simulink model "BRO_piston_MOD_test"  (R2020b)
settings: Solver=FixedStepAuto  StartTime=0.0  StopTime=time_max  FixedStep=.1  RelTol=1e-3
values from neighbouring files (symbols this model uses):
  A_mem = 30    [BRO_parameters_MOD.m]    (also in Copy_of_BRO_parameters_MOD.m; Large2.m = 29.6; Parameters_test2.m = 40.88; Small_Ref.m = 7.4)
  A_p = 0.25*pi*d_p^2    (= 0.00810731966556)    [BRO_parameters_MOD.m]    (also in Copy_of_BRO_parameters_MOD.m; Large2.m = 0.2105152; Parameters_test2.m = 1; Small_Ref.m = 0.03684016)
  A_w = 2/3600*1e-3    (= 5.55555555556e-07)    [BRO_parameters_MOD.m]    (also in Copy_of_BRO_parameters_MOD.m; Large2.m = 5.56e-12; Parameters_test2.m = 5.56e-07; Small_Ref.m = 5.56e-12)
  b = i*R*T*1e-2/M_NaCl*.93    (= 0.792350469684)    [BRO_parameters_MOD.m]    (also in Copy_of_BRO_parameters_MOD.m; Large2.m = 81215.9231426; Parameters_test2.m = 0.812159231426; Small_Ref.m = 81215.9231426)
  C_f_i = 35    [BRO_parameters_MOD.m]    (also in Copy_of_BRO_parameters_MOD.m; Large2.m; Parameters_test2.m; Small_Ref.m)
  D = 1.47e-9    (= 1.47e-09)    [BRO_parameters_MOD.m]    (also in Copy_of_BRO_parameters_MOD.m; Large2.m; Parameters_test2.m; Small_Ref.m)
  eta_cp = 0.65    [BRO_parameters_MOD.m]    (also in Copy_of_BRO_parameters_MOD.m; Large2.m; Parameters_test2.m; Small_Ref.m)
  eta_hp = 0.85    [BRO_parameters_MOD.m]    (also in Copy_of_BRO_parameters_MOD.m; Large2.m = 1; Parameters_test2.m; Small_Ref.m)
  L_mem = 0.96    [BRO_parameters_MOD.m]    (also in Copy_of_BRO_parameters_MOD.m; Large2.m; Parameters_test2.m = 1.016; Small_Ref.m)
  L_tank = 1    [Large2.m]    (also in Parameters_test2.m = 4.57856; Small_Ref.m)
  n_par = 5    [Large2.m]    (also in Parameters_test2.m = 2; Small_Ref.m = 14)
  n_ser = 4    [Large2.m]    (also in Parameters_test2.m; Small_Ref.m = 1)
  nu = 8.56e-7    (= 8.56e-07)    [BRO_parameters_MOD.m]    (also in Copy_of_BRO_parameters_MOD.m; Large2.m; Parameters_test2.m; Small_Ref.m)
  Q_cp = Q_p_des / RR_inst_des - Q_p_des    (= 0.04438224)    [Large2.m]    (also in Parameters_test2.m = 0.0015342264; Small_Ref.m = 0.007766892)
  rho_f = 1025    [BRO_parameters_MOD.m]    (also in Copy_of_BRO_parameters_MOD.m; Large2.m; Parameters_test2.m; Small_Ref.m)
  Sc = nu/D    (= 582.31292517)    [BRO_parameters_MOD.m]    (also in Copy_of_BRO_parameters_MOD.m; Large2.m; Parameters_test2.m; Small_Ref.m)
  thick = 7.112e-4    (= 0.0007112)    [Large2.m]    (also in Parameters_test2.m = 0.028; Small_Ref.m)
  V_D_hpp = 2.27e-6    (= 2.27e-06)    [Large2.m]    (also in Parameters_test2.m; Small_Ref.m)
  V_mem = A_mem*t/2    (= 0.010668)    [BRO_parameters_MOD.m]    (also in Copy_of_BRO_parameters_MOD.m; Large2.m = 0.01052576; Parameters_test2.m = 0.57232; Small_Ref.m = 0.00263144)
  V_tank_i = A_p*L_max    (= 0.00494222206813)    [BRO_parameters_MOD.m]    (also in Copy_of_BRO_parameters_MOD.m; Large2.m = 0.2105152; Parameters_test2.m = 4.57856; Small_Ref.m = 0.03684016)
libraries: simulink x2
settings Model: Creator=abhimanyu_das  LastModifiedBy=9alan
settings DebuggingCC: UnderSpecifiedDimensionMsg=warning

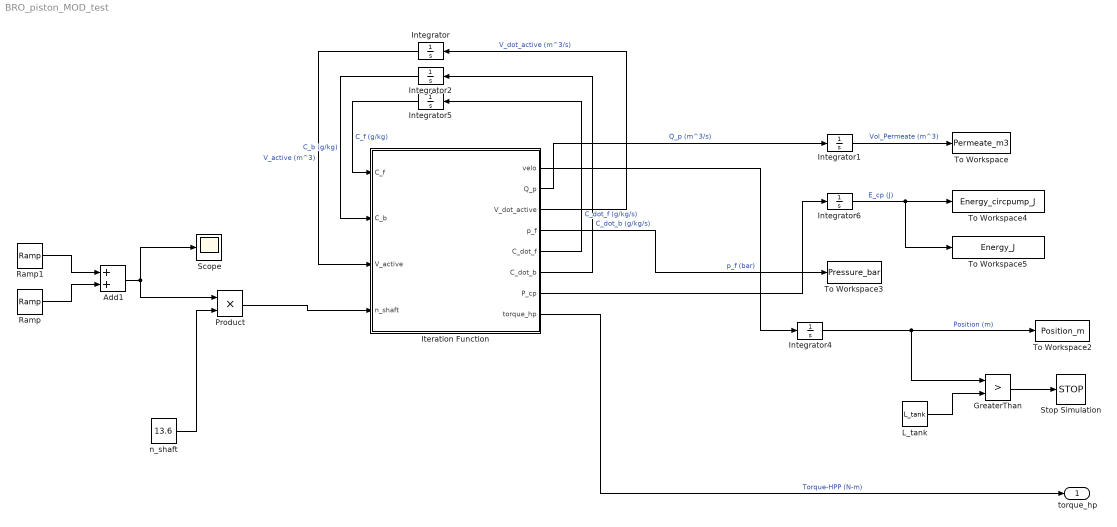
== system BRO_piston_MOD_test ==
  Add1 : Sum
  GreaterThan : RelationalOperator  Operator=>  OutDataTypeStr=boolean  RndMeth=Simplest
  Integrator : Integrator  InitialCondition=V_tank_i
  Integrator1 : Integrator  InitialCondition=0.001
  Integrator2 : Integrator  InitialCondition=C_f_i
  Integrator4 : Integrator  InitialCondition=0.001
  Integrator5 : Integrator  InitialCondition=C_f_i
  Integrator6 : Integrator  InitialCondition=0.001
  Iteration Function : MATLAB Function  TreatAsAtomicUnit=on
  L_tank : Constant  Value=L_tank
  Product : Product
  Ramp : simulink/Sources/Ramp  slope=-0.1  start=10  InitialOutput=0
  Ramp1 : simulink/Sources/Ramp  slope=0.1  start=0  InitialOutput=0
  Scope : Scope
  Stop Simulation : Stop
  To Workspace : ToWorkspace  VariableName=Permeate_m3  SaveFormat=Timeseries  SampleTime=-1
  To Workspace2 : ToWorkspace  VariableName=Position_m  SaveFormat=Timeseries  SampleTime=-1
  To Workspace3 : ToWorkspace  VariableName=Pressure_bar  SaveFormat=Timeseries  SampleTime=-1
  To Workspace4 : ToWorkspace  VariableName=Energy_circpump_J  SaveFormat=Timeseries  SampleTime=-1
  To Workspace5 : ToWorkspace  VariableName=Energy_J  SaveFormat=Timeseries  SampleTime=-1
  n_shaft : Constant  Value=13.6
  torque_hp : Outport
  wires:
  Iteration Function/3(V_dot_active) -> Integrator/1  "V_dot_active (m^3/s)"
  Integrator/1 -> Iteration Function/3(V_active)  "V_active (m^3)"
  Iteration Function/6(C_dot_b) -> Integrator2/1  "C_dot_b (g/kg/s)"
  Iteration Function/5(C_dot_f) -> Integrator5/1  "C_dot_f (g/kg/s)"
  Integrator5/1 -> Iteration Function/1(C_f)  "C_f (g/kg)"
  Iteration Function/4(p_f) -> To Workspace3/1  "p_f (bar)"
  Integrator1/1 -> To Workspace/1  "Vol_Permeate (m^3)"
  Iteration Function/1(velo) -> Integrator4/1
  Integrator4/1 -> GreaterThan/1, To Workspace2/1  "Position (m)"
  Integrator2/1 -> Iteration Function/2(C_b)  "C_b (g/kg)"
  Iteration Function/7(P_cp) -> Integrator6/1
  Integrator6/1 -> To Workspace5/1, To Workspace4/1  "E_cp (J)"
  Iteration Function/2(Q_p) -> Integrator1/1  "Q_p (m^3/s)"
  Iteration Function/8(torque_hp) -> torque_hp/1  "Torque-HPP (N-m)"
  Ramp1/1 -> Add1/1
  Ramp/1 -> Add1/2
  Add1/1 -> Scope/1, Product/1
  n_shaft/1 -> Product/2
  Product/1 -> Iteration Function/4(n_shaft)
  L_tank/1 -> GreaterThan/2
  GreaterThan/1 -> Stop Simulation/1

== matlab function BRO_piston_MOD_test/Iteration Function ==
  data: velo output; Q_p output; C_f input; C_b input; V_active input; V_dot_active output; p_f output; C_dot_f output; C_dot_b output; n_shaft input; P_cp output; torque_hp output; V_D_hpp parameter; eta_cp parameter; n_par parameter; n_ser parameter; L_mem parameter; A_mem parameter; V_mem parameter; A_w parameter; thick parameter; nu parameter; D parameter; Sc parameter; b parameter; rho_f parameter; eta_hp parameter; Q_cp parameter; A_p parameter
function [velo, Q_p, V_dot_active, p_f, C_dot_f, C_dot_b, P_cp, torque_hp] = Iteration_Function(C_f, C_b, V_active, n_shaft, V_D_hpp, eta_cp, n_par, n_ser, L_mem, A_mem, V_mem, A_w, thick, nu, D, Sc, b, rho_f, eta_hp, Q_cp, A_p)
%% CONTROL EFFORT

%% Pump Flow Rate Conversion
Q_hp = n_shaft * V_D_hpp;              %flow rate of HPP (assuming same shaft speed as HM) [m^3/s]

%% Flow Rates and Piston Velocity
Q_p = Q_hp;                        %Permeate flow rate [m^3/s]
Q_b = Q_cp;                        %Brine flow rate [m^3/s]
Q_f = Q_hp + Q_b;                  %Feed flow rate [m^3/s]
V_dot_active = Q_b - Q_f;          %Volumetric flow rate through the tank

velo = -(V_dot_active)/A_p;        %velocity of piston [m/s]

%% Salinity Dynamics 2
D_h = 2 * thick;
C_dot_f = (-Q_f * C_f + Q_b * C_b - C_f*V_dot_active)/V_active; 
C_dot_b = 2*(Q_f * C_f - Q_b * C_b)/(V_mem * n_par * n_ser) - C_dot_f;
Q_avg = (0.5/(n_par))*(Q_f + Q_b);              %Average flow rate on feed side [m^3/s]
u_avg = Q_avg*2*L_mem/(thick*A_mem);                      %Average velocity on feed side [m/s]
Re = u_avg * thick / nu;                                      %Reynolds number                     
f = 3.23*Re^-0.3;                                       %friction factor
p_drop = n_ser*f*L_mem*rho_f*u_avg^2/(2*D_h);                 %Pressure drop across a membrane module [bar]


J_w = Q_p/(A_mem*n_ser*n_par);                         %instantaneous flux [m/s]
Sh = .20*(Re^.57*Sc^.4);                                %Sherwood number  https://www.sciencedirect.com/science/article/pii/S0011916420313035?via%3Dihub
k = Sh*D/D_h;                                           %Mass transfer coefficient [m/s]
C_mem_avg = 0.5*(C_f+C_b);                                %Average bulk salinity on feed side [g/kg]

pi = b*C_mem_avg*exp(J_w/k);                              %Feed side osmotic pressure [bar]
p_f = J_w/A_w + pi;                                    %hi p pump pressure [bar] *******   

%% Torque and Power Calculation
% P_hp = Q_hp*p_in*1e5/eta_hp;            %high pressure pump power consumption [W]
P_cp = Q_cp*p_drop*1e5/eta_cp;          %circulation pump power consumption [W]
torque_hp = (V_D_hpp * p_f) / eta_hp;        %torque generated by HPP
